simulink model "manipulator_sim"  (R2015b)
settings: Solver=VariableStepAuto  StartTime=0.0  StopTime=70  RelTol=1e-3
values from neighbouring files (symbols this model uses):
  c1 = m*g*L/I    (= 1)    [ManipulatorMain.m]
  c2 = k/I    (= 1)    [ManipulatorMain.m]
  c3 = k^2/(I*J)    (= 1)    [ManipulatorMain.m]
  c4 = k/(I*J)    (= 1)    [ManipulatorMain.m]
  c5 = k/J    (= 1)    [ManipulatorMain.m]
  J = 1    [ManipulatorMain.m]    (also in sampleit.m)
  k = 1    [ManipulatorMain.m]    (also in sampleit.m = 200)
  K_manip = lqr(A_manip,B_manip,eye(4),1*eye(1),[])    [ManipulatorMain.m]
  L = 1    [ManipulatorMain.m]    (also in sampleit.m)
  u_max = 10    [ManipulatorMain.m]
  u_min = -10    [ManipulatorMain.m]
  x1_m_0 = -pi/10    (= -0.314159265359)    [ManipulatorMain.m]
  x2_m_0 = 0    [ManipulatorMain.m]
  x3_m_0 = +pi/10    (= 0.314159265359)    [ManipulatorMain.m]
  x4_m_0 = 0    [ManipulatorMain.m]
settings Model: Creator=mlab-retro  LastModifiedBy=mlab-retro

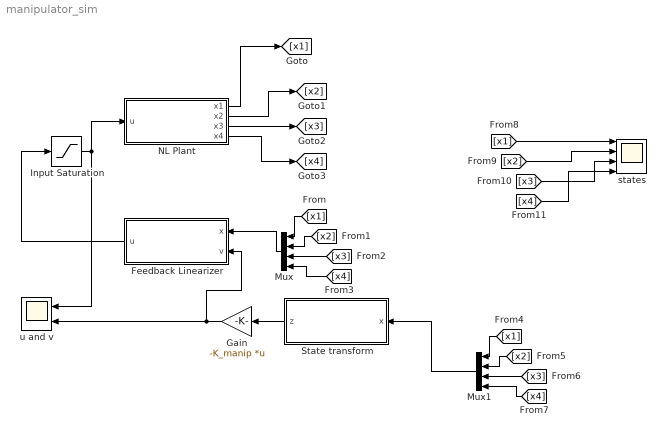
== system manipulator_sim ==
  Feedback Linearizer : Subsystem
  Gain : Gain  Gain=-K_manip  Multiplication=Matrix(K*u) (u vector)
  Input Saturation : Saturate  UpperLimit=u_max  LowerLimit=u_min  LinearizeAsGain=off
  Mux : Mux
  Mux1 : Mux
  NL Plant : Subsystem
  State transform : Subsystem
  states : Scope  NumInputPorts=4
  u and v : Scope  NumInputPorts=2
  wires:
  Mux/1 -> Feedback Linearizer/1(x)
  Mux1/1 -> State transform/1(x)
  State transform/1(z) -> Gain/1
  Gain/1 -> Feedback Linearizer/2(v), u and v/2
  Feedback Linearizer/1(u) -> Input Saturation/1
  Input Saturation/1 -> u and v/1, NL Plant/1(u)
  NL Plant/1(x1) -> [x1]
  NL Plant/2(x2) -> [x2]
  NL Plant/3(x3) -> [x3]
  NL Plant/4(x4) -> [x4]
  [x1] -> Mux/1
  [x2] -> Mux/2
  [x3] -> Mux/3
  [x4] -> Mux/4
  [x1] -> Mux1/1
  [x2] -> Mux1/2
  [x3] -> Mux1/3
  [x4] -> Mux1/4
  [x1] -> states/1
  [x2] -> states/2
  [x3] -> states/3
  [x4] -> states/4

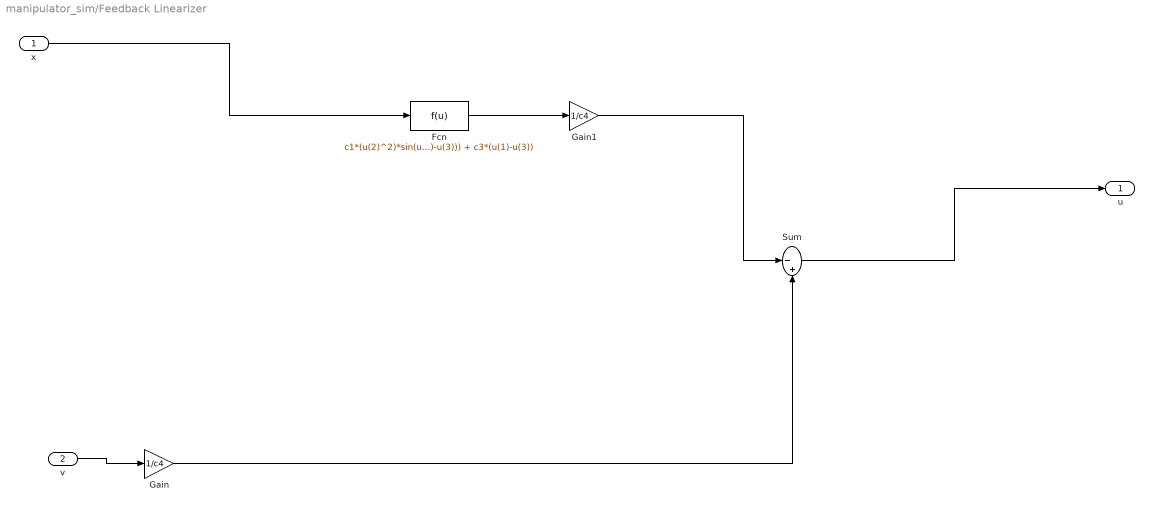
== system manipulator_sim/Feedback Linearizer ==
  x : Inport
  v : Inport  Port=2
  Fcn : Fcn  Expr=c1*(u(2)^2)*sin(u(1)) - (c1*cos(u(1))-c2)*(c1*sin(u(1))+c2*(u(1)-u(3))) + c3*(u(1)-u(3))
  Gain : Gain  Gain=1/c4
  Gain1 : Gain  Gain=1/c4
  Sum : Sum  Inputs=|-+
  u : Outport
  wires:
  v/1 -> Gain/1
  x/1 -> Fcn/1
  Fcn/1 -> Gain1/1
  Gain/1 -> Sum/2
  Gain1/1 -> Sum/1
  Sum/1 -> u/1

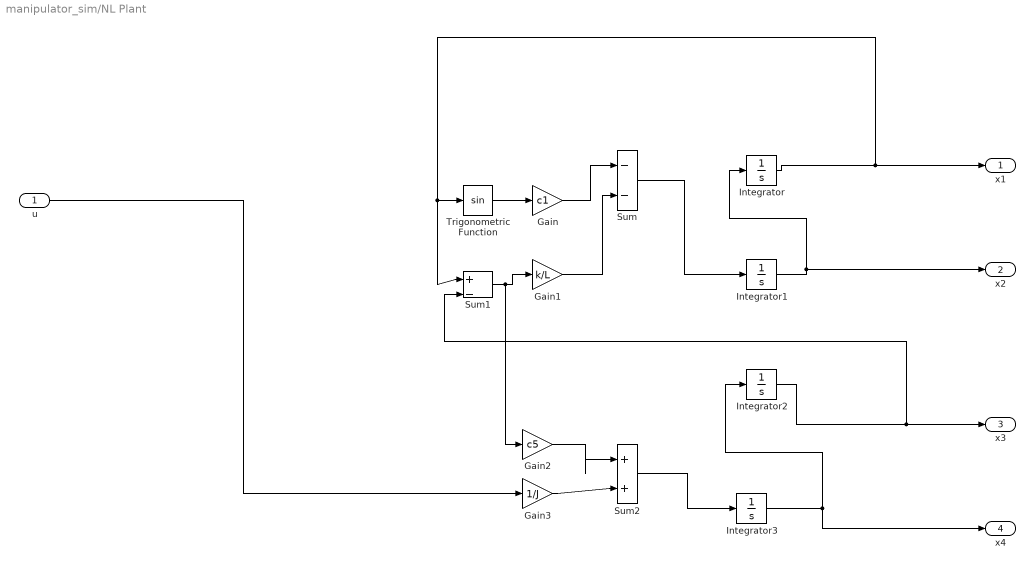
== system manipulator_sim/NL Plant ==
  u : Inport
  Gain : Gain  Gain=c1
  Gain1 : Gain  Gain=k/L
  Gain2 : Gain  Gain=c5
  Gain3 : Gain  Gain=1/J
  Integrator : Integrator  InitialCondition=x1_m_0
  Integrator1 : Integrator  InitialCondition=x2_m_0
  Integrator2 : Integrator  InitialCondition=x3_m_0
  Integrator3 : Integrator  InitialCondition=x4_m_0
  Sum : Sum  Inputs=|--
  Sum1 : Sum  Inputs=|+-
  Sum2 : Sum  Inputs=|++
  Trigonometric Function : Trigonometry
  x1 : Outport
  x2 : Outport  Port=2
  x3 : Outport  Port=3
  x4 : Outport  Port=4
  wires:
  Integrator/1 -> Sum1/1, Trigonometric Function/1, x1/1
  Integrator1/1 -> Integrator/1, x2/1
  Integrator2/1 -> Sum1/2, x3/1
  Integrator3/1 -> Integrator2/1, x4/1
  Trigonometric Function/1 -> Gain/1
  Gain/1 -> Sum/1
  Sum/1 -> Integrator1/1
  Sum1/1 -> Gain2/1, Gain1/1
  Gain1/1 -> Sum/2
  Gain2/1 -> Sum2/1
  Sum2/1 -> Integrator3/1
  Gain3/1 -> Sum2/2
  u/1 -> Gain3/1

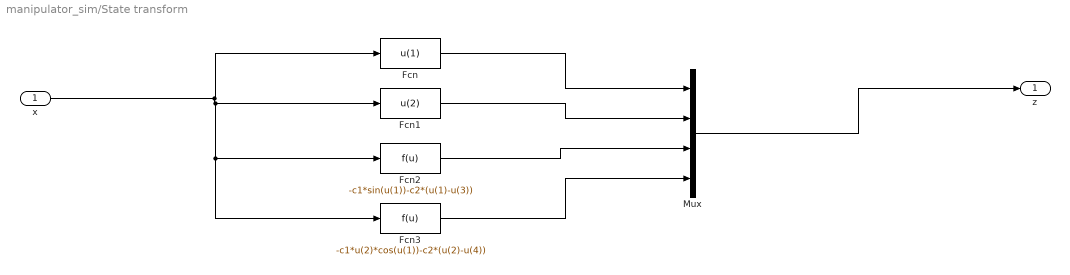
== system manipulator_sim/State transform ==
  x : Inport
  Fcn : Fcn  Expr=u(1)
  Fcn1 : Fcn  Expr=u(2)
  Fcn2 : Fcn  Expr=-c1*sin(u(1))-c2*(u(1)-u(3))
  Fcn3 : Fcn  Expr=-c1*u(2)*cos(u(1))-c2*(u(2)-u(4))
  Mux : Mux
  z : Outport
  wires:
  Mux/1 -> z/1
  x/1 -> Fcn3/1, Fcn2/1, Fcn1/1, Fcn/1
  Fcn/1 -> Mux/1
  Fcn1/1 -> Mux/2
  Fcn2/1 -> Mux/3
  Fcn3/1 -> Mux/4
